simulink model "ms2"  (R2023b)
settings: Solver=VariableStepAuto  StartTime=0.0  StopTime=10.0  RelTol=1e-3
undefined symbols (not defined in the file): A, F, J, L, P, R, Vf
settings Model: Creator=lylia  LastModifiedBy=lylia

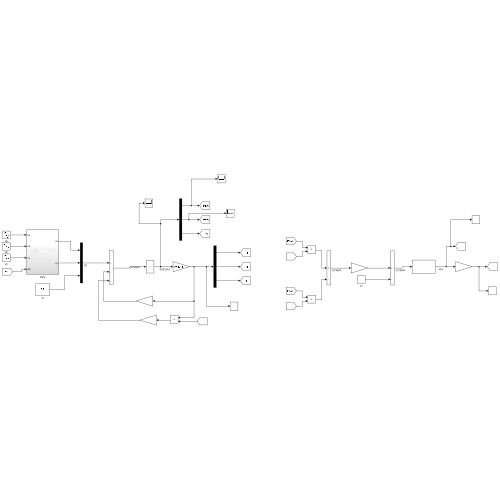
[thumbnail: Simulink's stored preview of the top-level diagram]
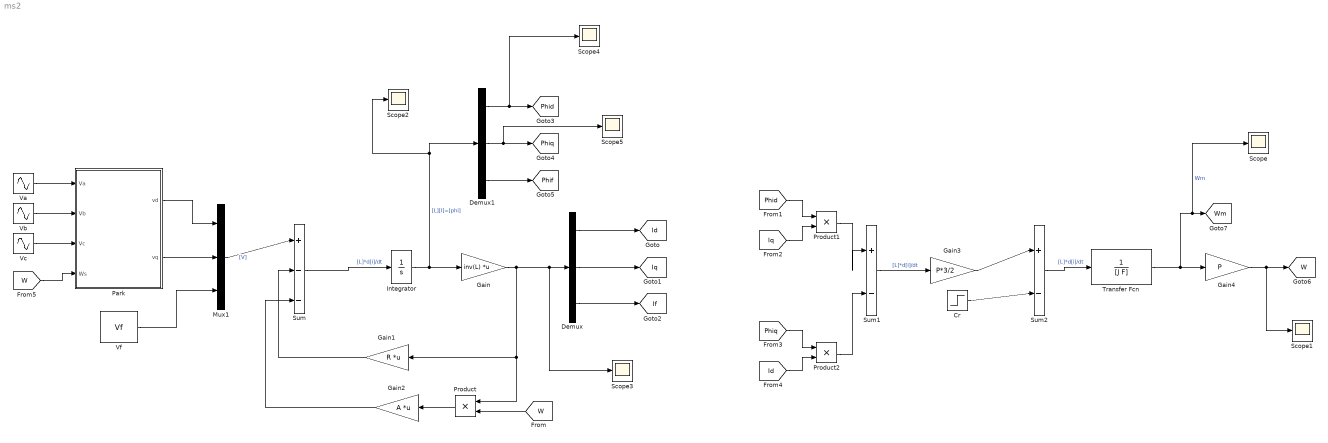
== system ms2 ==
  Cr : Step  Time=2  Before=0.5  After=5  SampleTime=0
  Demux : Demux  Outputs=3
  Demux1 : Demux  Outputs=3
  Gain : Gain  Gain=inv(L)  Multiplication=Matrix(K*u)
  Gain1 : Gain  Gain=R  Multiplication=Matrix(K*u)
  Gain2 : Gain  Gain=A  Multiplication=Matrix(K*u)
  Gain3 : Gain  Gain=P*3/2
  Gain4 : Gain  Gain=P
  Integrator : Integrator
  Mux1 : Mux  Inputs=3
  Park : Subsystem
  Product : Product
  Product1 : Product
  Product2 : Product
  Scope{,1..5} (6 alike) : Scope
  Sum : Sum  Inputs=|+--
  Sum1 : Sum  Inputs=|+-
  Sum2 : Sum  Inputs=|+-
  Transfer Fcn : TransferFcn  Denominator=[J F]
  Va : Sin  Amplitude=220*sqrt(2)  Frequency=2*pi*50  SampleTime=0
  Vb : Sin  Amplitude=220*sqrt(2)  Frequency=2*pi*50  Phase=-2*pi/3  SampleTime=0
  Vc : Sin  Amplitude=220*sqrt(2)  Frequency=2*pi*50  Phase=2*pi/3  SampleTime=0
  Vf : Constant  Value=Vf
  tag scope: Id=global, If=global, Iq=global, Phid=global, Phif=global, Phiq=global, W=global, Wm=global
  wires:
  [Phid] -> Product1/1
  Park/1(vd) -> Mux1/1
  Demux1/1 -> Scope4/1, [Phid]
  Cr/1 -> Sum2/2
  Sum2/1 -> Transfer Fcn/1  "[L]*d[i]/dt"
  [Phiq] -> Product2/1
  Demux/1 -> [Id]
  Sum1/1 -> Gain3/1  "[L]*d[i]/dt"
  [Iq] -> Product1/2
  Demux1/2 -> Scope5/1, [Phiq]
  Gain3/1 -> Sum2/1
  Product2/1 -> Sum1/2
  Demux1/3 -> [Phif]
  Product1/1 -> Sum1/1
  Vc/1 -> Park/3(Vc)
  Gain2/1 -> Sum/3
  Demux/3 -> [If]
  Gain/1 -> Scope3/1, Demux/1, Product/1, Gain1/1
  Sum/1 -> Integrator/1  "[L]*d[i]/dt"
  Gain4/1 -> Scope1/1, [W]
  Integrator/1 -> Scope2/1, Demux1/1, Gain/1  "[L][I]=[phi]"
  [W] -> Park/4(Ws)
  [W] -> Product/2
  Demux/2 -> [Iq]
  Gain1/1 -> Sum/2
  Vf/1 -> Mux1/3
  [Id] -> Product2/2
  Mux1/1 -> Sum/1  "[V]"
  Va/1 -> Park/1(Va)
  Product/1 -> Gain2/1
  Vb/1 -> Park/2(Vb)
  Park/2(vq) -> Mux1/2
  Transfer Fcn/1 -> Scope/1, [Wm], Gain4/1  "Wm"

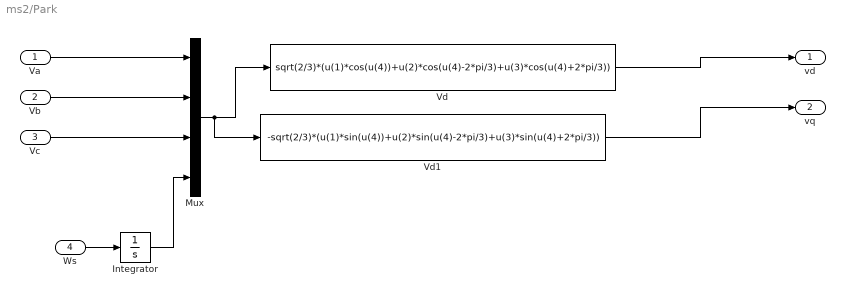
== system ms2/Park ==
  Va : Inport
  Vb : Inport  Port=2
  Vc : Inport  Port=3
  Ws : Inport  Port=4
  Integrator : Integrator
  Mux : Mux
  Vd : Fcn  Expr=sqrt(2/3)*(u(1)*cos(u(4))+u(2)*cos(u(4)-2*pi/3)+u(3)*cos(u(4)+2*pi/3))
  Vd1 : Fcn  Expr=-sqrt(2/3)*(u(1)*sin(u(4))+u(2)*sin(u(4)-2*pi/3)+u(3)*sin(u(4)+2*pi/3))
  vd : Outport
  vq : Outport  Port=2
  wires:
  Vc/1 -> Mux/3
  Integrator/1 -> Mux/4
  Vb/1 -> Mux/2
  Vd/1 -> vd/1
  Mux/1 -> Vd1/1, Vd/1
  Va/1 -> Mux/1
  Ws/1 -> Integrator/1
  Vd1/1 -> vq/1
